simulink model "Wiper_rev_01_00_student"  (R2021b)
settings: Solver=FixedStepDiscrete  StartTime=0.0  StopTime=30  FixedStep=0.25  RelTol=1e-3
undefined symbols (not defined in the file): sigbuilder_block
settings Model: Creator=matlab01  LastModifiedBy=user
settings SolverCC: AlgebraicLoopSolver=TrustRegion
settings DebuggingCC: SFMachineParentedDataDiag=warning

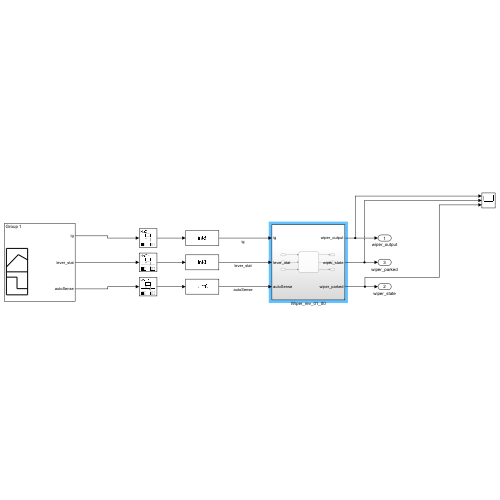
[thumbnail: Simulink's stored preview of the top-level diagram]
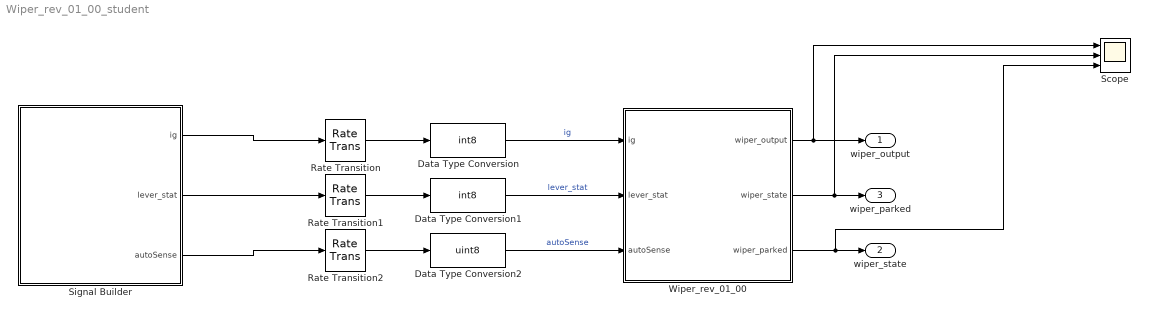
== system Wiper_rev_01_00_student ==
  Data Type Conversion : DataTypeConversion  OutDataTypeStr=int8
  Data Type Conversion1 : DataTypeConversion  OutDataTypeStr=int8
  Data Type Conversion2 : DataTypeConversion  OutDataTypeStr=uint8
  Rate Transition : RateTransition
  Rate Transition1 : RateTransition
  Rate Transition2 : RateTransition
  Scope : Scope  NumInputPorts=3
  Signal Builder : Subsystem  Tag=STV Subsys  LoadFcn=sigbuilder_block('load');  StartFcn=sigbuilder_block('start');  StopFcn=sigbuilder_block('stop');  ClipboardFcn=sigbuilder_block('clipboard');  mask(Sigbuilder block){tuvar=[0:10]}
      mask help: Simulink:masks:SigbuilderBlock_MD
      mask init:
      | if ~strcmp(get_param(bdroot(gcbh),'SimulationStatus'),'stopped') tuvar = sigbuilder_block('maskInit'); end
      settings: CopyFcn=sigbuilder_block('copy');  DeleteFcn=sigbuilder_block('delete');  ModelCloseFcn=sigbuilder_block('modelClose');  PreSaveFcn=sigbuilder_block('preSave');  PauseFcn=sigbuilder_block('pause');  ContinueFcn=sigbuilder_block('continue');  NameChangeFcn=sigbuilder_block('namechange');  OpenFcn=sigbuilder_block('open',[222 42.6 550.8 496.8 ]);  CloseFcn=sigbuilder_block('close');
      mask Display: plot(0, 0, 100, 100,[2, 2, 32, 32, 2], [68, 8, 8, 68, 68],[32, 2], [38, 38], [32, 19, 2],[53, 60, 44], [32, 17, 17, 2],[16, 16, 31, 31]);txt = getActiveGroup(gcbh);text(2, 100, txt,'verticalAlignment', 'top');
  Wiper_rev_01_00 : Subsystem
  wiper_output : Outport
  wiper_state : Outport  Port=2
  wiper_parked : Outport  Port=3
  wires:
  Data Type Conversion/1 -> Wiper_rev_01_00/1(ig)  "ig"
  Data Type Conversion1/1 -> Wiper_rev_01_00/2(lever_stat)  "lever_stat"
  Data Type Conversion2/1 -> Wiper_rev_01_00/3(autoSense)  "autoSense"
  Rate Transition/1 -> Data Type Conversion/1
  Rate Transition2/1 -> Data Type Conversion2/1
  Rate Transition1/1 -> Data Type Conversion1/1
  Wiper_rev_01_00/1(wiper_output) -> Scope/1, wiper_output/1
  Wiper_rev_01_00/2(wiper_state) -> Scope/2, wiper_parked/1
  Wiper_rev_01_00/3(wiper_parked) -> Scope/3, wiper_state/1
  Signal Builder/1(ig) -> Rate Transition/1
  Signal Builder/2(lever_stat) -> Rate Transition1/1
  Signal Builder/3(autoSense) -> Rate Transition2/1

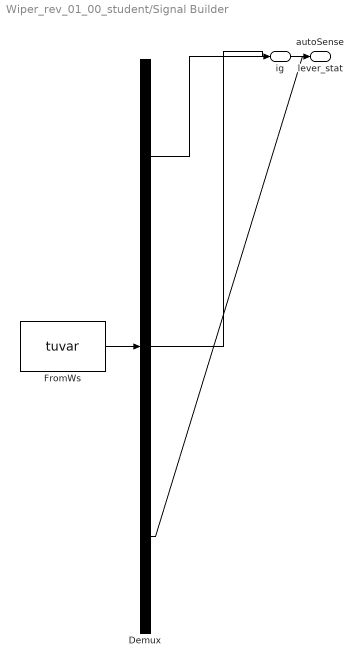
== system Wiper_rev_01_00_student/Signal Builder ==
  Demux : Demux  Tag=STV Demux  Outputs=3
      settings: DisplayOption=none
  FromWs : FromWorkspace  Tag=STV FromWs  VariableName=tuvar
      SigBuilderData=|
      | common.afterFinalStr = 'Extrapolate'
      | common.sampleTime = 0
      | dataSet.timeRange = [0 10]
      | dataSet.name = 'Group 1'
      | sbobj.Groups.Name = 'Group 1'
      | sbobj.Groups.Signals(1).Name = 'ig'
      | sbobj.Groups.Signals(1).XData = [0 1 1 9 9 10]
      | sbobj.Groups.Signals(1).YData = [0 0 1 1 0 0]
      | sbobj.Groups.Signals(2).Name = 'lever_stat'
      | sbobj.Groups.Signals(2).XData = [0 2 2 3 3 4 4 5 5 6 6 7 7 8 8 9 9 10]
      | sbobj.Groups.Signals(2).YData = [0 0 -1 -1 0 0 1 1 2 2 3 3 2 2 0.95 1 0 -0.05]
      | sbobj.Groups.Signals(3).Name = 'autoSense'
      | sbobj.Groups.Signals(3).XData = [0 4 4 4.5 4.5 5 5 8 8 9 9 10]
      | sbobj.Groups.Signals(3).YData = [0 0 1 1 2 2 0 0 2 2 0 0]
  ig : Outport  Tag=STV Outport
  lever_stat : Outport  Tag=STV Outport  Port=2
  autoSense : Outport  Tag=STV Outport  Port=3
  wires:
  Demux/1 -> ig/1
  FromWs/1 -> Demux/1
  Demux/2 -> lever_stat/1
  Demux/3 -> autoSense/1

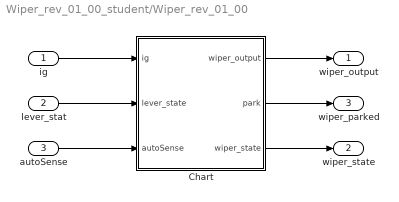
== system Wiper_rev_01_00_student/Wiper_rev_01_00 ==
  ig : Inport
  lever_stat : Inport  Port=2
  autoSense : Inport  Port=3
  Chart : Stateflow chart  TreatAsAtomicUnit=on
  wiper_output : Outport
  wiper_state : Outport  Port=2
  wiper_parked : Outport  Port=3
  wires:
  ig/1 -> Chart/1(ig)
  lever_stat/1 -> Chart/2(lever_state)
  autoSense/1 -> Chart/3(autoSense)
  Chart/1(wiper_output) -> wiper_output/1
  Chart/2(park) -> wiper_parked/1
  Chart/3(wiper_state) -> wiper_state/1

== stateflow chart Wiper_rev_01_00_student/Wiper_rev_01_00/Chart ==
  state Mist
    en:
    wiper_state = MIST;
    du:
    wiper_output = ON
    exit:
    park = ON;
    wiper_output = OFF;
  state Wiper_off
    en:
    wiper_state = OFF;
    park = ON;
    du:
    wiper_state = OFF;
    exit:
    park = OFF;
  state Auto
    en:
    wiper_state = AUTO;
    du:
    wiper_output = ON;
    exit:
    wiper_output = OFF;
  state Lo
    en:
    wiper_state = LO;
    du:
    wiper_output = ON;
    exit:
    wiper_output = OFF;
  state Hi
    wiper_state = HI;
    du:
    wiper_output = ON;
    exit:
    wiper_output = OFF;
  (default) -> Wiper_off : {wiper_output = OFF}
  Wiper_off -> Mist [order 1] : [lever_state== MIST&&ig==ON]
  Mist -> Wiper_off [order 1] : [lever_state == OFF&&ig==ON]
  (junction 76) -> Wiper_off
  Auto -> Wiper_off [order 1] : [lever_state==OFF&&ig==ON]
  Wiper_off -> Auto [order 2] : [lever_state==AUTO&&ig==ON]
  Mist -> (junction 76) [order 2] : [ig==OFF]
  Auto -> (junction 76) [order 3] : [ig==OFF]
  Lo -> (junction 76) [order 3] : [ig==OFF]
  Hi -> (junction 76) [order 2] : [ig==OFF]
  Lo -> Auto [order 1] : [lever_state==AUTO&&ig==ON]
  Auto -> Lo [order 2] : [lever_state==LO&&ig==ON]
  Lo -> Hi [order 2] : [lever_state==HI&&ig==ON]
  Hi -> Lo [order 1] : [lever_state==LO&&ig==ON]
  data: ig input int8; lever_state input int8; autoSense input uint8; wiper_output output int8; park output int8; AUTO constant int8 =1; wiper_state output int8; HI constant int8 =3; LO constant int8 =2; MIST constant int8 =-1; OFF constant int8 =0; ON constant int8 =1
